simulink model "SimulinkBlocks"  (R2024b)
settings: Solver=VariableStepAuto  StartTime=0.0  StopTime=NCS.simTime  FixedStep=Td  RelTol=1e-3
InitFcn:
  | set_param(gcs, 'SimulationCommand', 'update')
undefined symbols (not defined in the file or in its folder): NCS, sfunchk
libraries: cstblocks x1, truetime x1
settings Model: Creator=jakob_ludwiger  LastModifiedBy=kala
settings SolverCC: AlgebraicLoopSolver=TrustRegion
settings DataIOCC: ReturnWorkspaceOutputs=off
settings DebuggingCC: UnconnectedInputMsg=warning  UnconnectedOutputMsg=warning  UnconnectedLineMsg=warning  ArithmeticOperatorsInVariantConditions=warning
settings ModelReferenceCC: EnableRefExpFcnMdlSchedulingChecks=on
settings SFSimCC: SimUseLocalCustomCode=off  CustomCodeUndefinedFunction=UseInterfaceOnly
settings RTWCC: RTWUseLocalCustomCode=off  GPUComputeCapability=3.5  DLArmComputeVersion=19.05
settings CodeAppCC: StateflowObjectComments=on

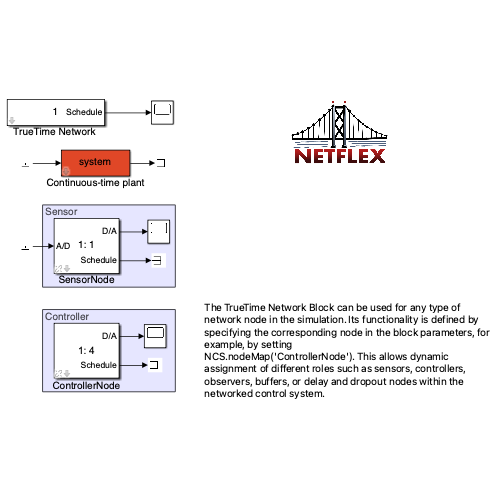
[thumbnail: Simulink's stored preview of the top-level diagram]
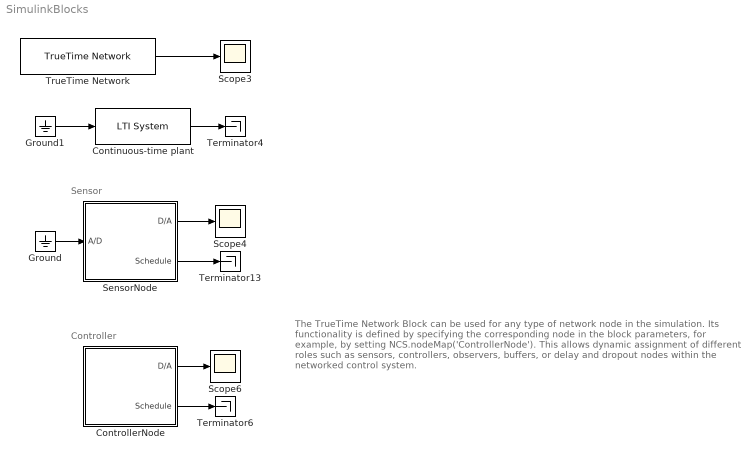
== system SimulinkBlocks ==
  note: The TrueTime Network Block can be used for any type of network node in the simulation. Its functionality is defined by specifying the corresponding node in the block parameters, for example, by setting
      | NCS.nodeMap('ControllerNode'). This allows dynamic assignment of different roles such as sensors, controllers, observers, buffers, or delay and dropout nodes within the networked control system.
  note: Sensor
  note: Controller
  Continuous-time plant : cstblocks/LTI System  sys=system  IC=initialState  PadeOrder=0
  ControllerNode : Subsystem  AncestorBlock=truetime/TrueTime Kernel  InitFcn=sfunchk(get_param(gcb,'sfun'));  mask{nodeObj=NCS.nodeMap('ControllerNode'), sfun=initFctWrapper, ntriggers=0, trigtype=falling, clockoffsetdrift=[0 0], schedoutput=on, battery=off, poweroutput=off, label=1: 4}
      mask prompts: nodeObj "Node Object"; sfun "Name of init function (MEX or MATLAB):"; ntriggers "Number of external triggers:"; trigtype "Trigger type:"; clockoffsetdrift "Local clock offset and drift:"; schedoutput "Show Schedule output port"; battery "Show Energy supply input port"; poweroutput "Show Power consumption output port"
      mask init:
      | set_param(gcb,'sfun', nodeObj.initFunctionWrapper)
      | %set_param(gcb,'args', [3 2])
      | args = nodeObj;
      | ninputsoutputs = [nodeObj.nIn nodeObj.nOut];
      | nwnodenbr = nodeObj.nodeNr;
      | ttkernel_callback(gcb,{sfun,args,ninputsoutputs,ntriggers,trigtype,nwnodenbr,clockoffsetdrift,schedoutput,battery,poweroutput})
      settings: ErrorFcn=ttkernel_error
      mask TypeOptions trigtype: rising | falling | either
      mask Display: disp(get_param(gcb,'label'))
  Ground : Ground
  Ground1 : Ground
  Scope3 : Scope
  Scope4 : Scope
  Scope6 : Scope
  SensorNode : Subsystem  AncestorBlock=truetime/TrueTime Kernel  InitFcn=sfunchk(get_param(gcb,'sfun'));  mask{nodeObj=NCS.nodeMap('SensorNode'), sfun=initFctWrapper, ntriggers=0, trigtype=falling, clockoffsetdrift=[0 0], schedoutput=on, battery=off, poweroutput=off, label=1: 1}
      mask prompts: nodeObj "Node Object"; sfun "Name of init function (MEX or MATLAB):"; ntriggers "Number of external triggers:"; trigtype "Trigger type:"; clockoffsetdrift "Local clock offset and drift:"; schedoutput "Show Schedule output port"; battery "Show Energy supply input port"; poweroutput "Show Power consumption output port"
      mask init: same as SimulinkBlocks/ControllerNode
      settings: ErrorFcn=ttkernel_error
      mask TypeOptions trigtype: rising | falling | either
      mask Display: disp(get_param(gcb,'label'))
  Terminator13 : Terminator
  Terminator4 : Terminator
  Terminator6 : Terminator
  "TrueTime Network " : truetime/TrueTime Network  nwtype=CSMA/CD (Ethernet)  nwnbr=1  nnodes=NCS.getMaxNodeNr  rate=1e8  minsize=200  lossprob=0  seed=0  bandwidths=[0.5 0.5]  slotsize=512  schedule=[1 1 2]  memsize=80000  buftype=Common buffer  overflow=Retransmit  dynSchedule=0  miniSlotSize=0  NIT=0  QSortMode=FIFO  sync=0  irtSchedule=0  nrtLength=0  nodeGraph=0  scheduleoutput=on
  wires:
  "TrueTime Network "/1 -> Scope3/1
  SensorNode/1(D/A) -> Scope4/1
  Ground/1 -> SensorNode/1(A/D)
  SensorNode/2(Schedule) -> Terminator13/1
  Ground1/1 -> Continuous-time plant/1
  Continuous-time plant/1 -> Terminator4/1
  ControllerNode/2(Schedule) -> Terminator6/1
  ControllerNode/1(D/A) -> Scope6/1

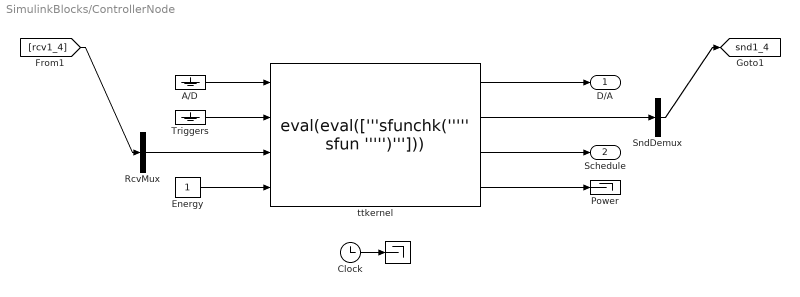
== system SimulinkBlocks/ControllerNode ==
  " " : Terminator
  A/D : Ground
  Clock : Clock
  Energy : Constant
  Power : Terminator
  RcvMux : Mux  Inputs=1
  SndDemux : Demux  Outputs=1
      settings: DisplayOption=none
  Triggers : Ground
  ttkernel : S-Function  FunctionName=eval(eval(['''sfunchk(''''' sfun ''''')''']))  Parameters=sfun, args, ninputsoutputs, ntriggers, trigtype, nwnodenbr, clockoffsetdrift  SFunctionDeploymentMode=off  EnableBusSupport=off
  D/A : Outport
  Schedule : Outport  Port=2
  tag scope: snd1_4=global
  wires:
  ttkernel/4 -> Power/1
  Energy/1 -> ttkernel/4
  A/D/1 -> ttkernel/1
  ttkernel/2 -> SndDemux/1
  ttkernel/1 -> D/A/1
  ttkernel/3 -> Schedule/1
  Triggers/1 -> ttkernel/2
  RcvMux/1 -> ttkernel/3
  Clock/1 -> " "/1
  [rcv1_4] -> RcvMux/1
  SndDemux/1 -> [snd1_4]

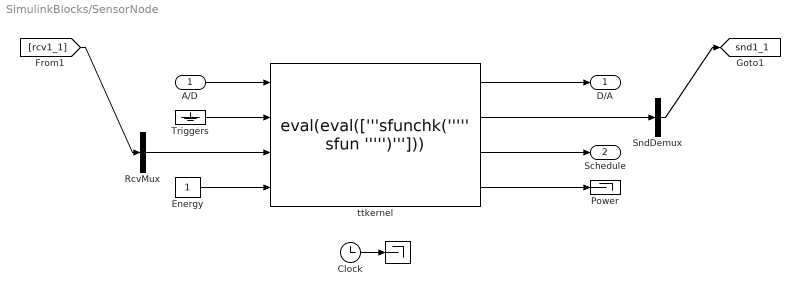
== system SimulinkBlocks/SensorNode ==
  A/D : Inport
  " " : Terminator
  Clock : Clock
  Energy : Constant
  Power : Terminator
  RcvMux : Mux  Inputs=1
  SndDemux : Demux  Outputs=1
      settings: DisplayOption=none
  Triggers : Ground
  ttkernel : S-Function  FunctionName=eval(eval(['''sfunchk(''''' sfun ''''')''']))  Parameters=sfun, args, ninputsoutputs, ntriggers, trigtype, nwnodenbr, clockoffsetdrift  SFunctionDeploymentMode=off  EnableBusSupport=off
  D/A : Outport
  Schedule : Outport  Port=2
  tag scope: snd1_1=global
  wires:
  Clock/1 -> " "/1
  RcvMux/1 -> ttkernel/3
  Triggers/1 -> ttkernel/2
  ttkernel/3 -> Schedule/1
  ttkernel/1 -> D/A/1
  ttkernel/2 -> SndDemux/1
  A/D/1 -> ttkernel/1
  Energy/1 -> ttkernel/4
  ttkernel/4 -> Power/1
  [rcv1_1] -> RcvMux/1
  SndDemux/1 -> [snd1_1]
